simulink model "arduino_run"  (R2022a)
settings: Solver=FixedStepAuto  StartTime=0.0  StopTime=100  RelTol=1e-3  EnableMultiTasking=on
model workspace: external: MATLAB File D:\personal_projects\robot\biped-robot\robot_DataFile2.m (data not in the file)
libraries: arduinolib x48, simulink x12
settings Model: ExtModeTrigDuration=2  Creator=isamu  LastModifiedBy=isamu
settings OptimizationCC: EnhancedBackFolding=on  PassReuseOutputArgsAs=Individual arguments  ZeroExternalMemoryAtStartup=off  ZeroInternalMemoryAtStartup=off  MaxStackSize=64  OptimizeBlockOrder=speed  DifferentSizesBufferReuse=on  OptimizationCustomize=off  EfficientTunableParamExpr=on
settings DebuggingCC: ParameterTunabilityLossMsg=error
settings HardwareCC: ProdBitPerInt=16  ProdBitPerPointer=16  ProdBitPerSizeT=16  ProdBitPerPtrDiffT=16  ProdLargestAtomicFloat=None  ProdWordSize=8  ProdHWDeviceType=Atmel->AVR  UseEmbeddedCoderFeatures=off  UseSimulinkCoderFeatures=off
settings SFSimCC: MATLABDynamicMemAlloc=off
settings RTWCC: SystemTargetFile=ert.tlc  HardwareBoard=Arduino Mega 2560  TemplateMakefile=ert_default_tmf  Toolchain=Arduino AVR  BuildConfiguration=Faster Runs
settings CodeAppCC: ForceParamTrailComments=on  IgnoreCustomStorageClasses=off  OperatorAnnotations=on  SimulinkDataObjDesc=on  SFDataObjDesc=on  InsertBlockDesc=on
settings ERTTargetCC: SupportContinuousTime=on  SupportNonInlinedSFcns=on  SupportVariableSizeSignals=on  ExtModeTransport=3  ExtModeStaticAlloc=on  ExtModeStaticAllocSize=2048  ExtModeMexFile=ext_xcp  ExtModeIntrfLevel=Level2 - Open

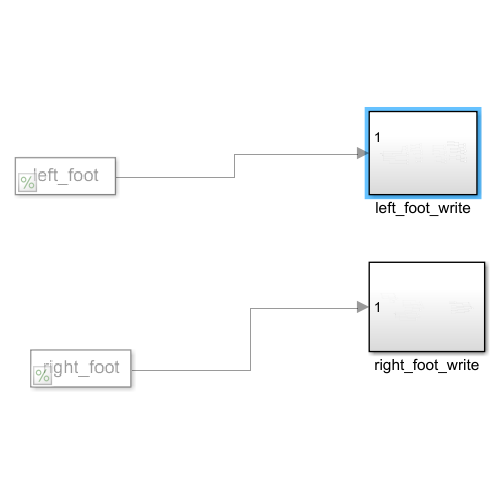
[thumbnail: Simulink's stored preview of the top-level diagram]
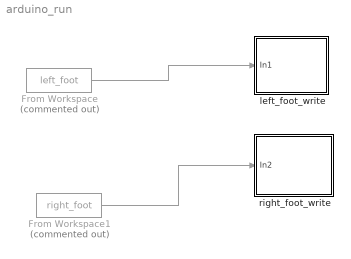
== system arduino_run ==
  From Workspace : FromWorkspace  Commented=on  VariableName=left_foot  OutDataTypeStr=Bus: left_foot_bus  SampleTime=0.045  OutputAfterFinalValue=Holding final value
  From Workspace1 : FromWorkspace  Commented=on  VariableName=right_foot  OutDataTypeStr=Bus: right_foot_bus  SampleTime=0.045  OutputAfterFinalValue=Holding final value
  left_foot_write : Subsystem
  right_foot_write : Subsystem
  wires:
  From Workspace/1 -> left_foot_write/1(In1)
  From Workspace1/1 -> right_foot_write/1(In2)

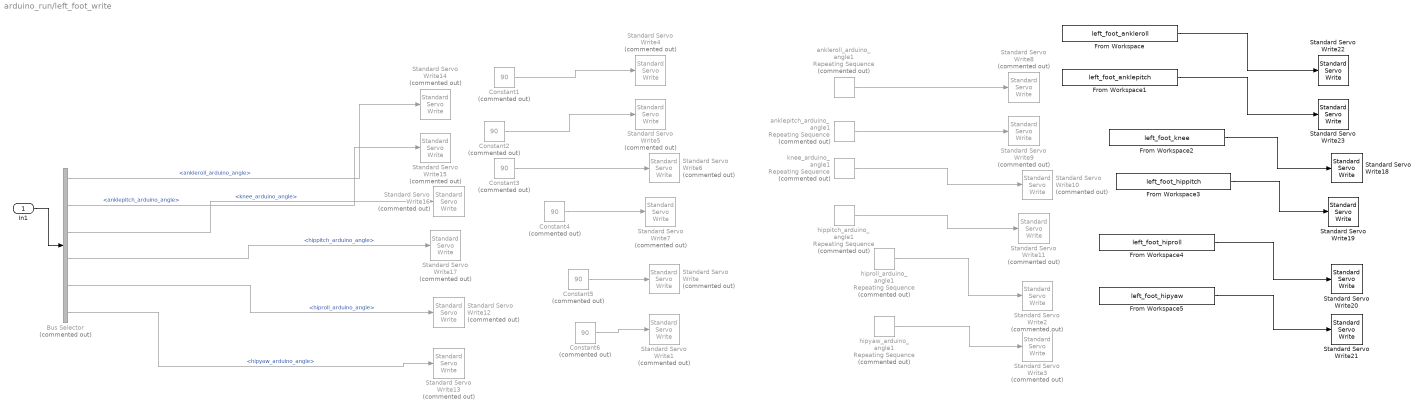
== system arduino_run/left_foot_write ==
  In1 : Inport
  Bus Selector : BusSelector  Commented=on  OutputSignals=ankleroll_arduino_angle,anklepitch_arduino_angle,knee_arduino_angle,hippitch_arduino_angle,hiproll_arduino_angle,hipyaw_arduino_angle
  Constant{1..6} (6 alike) : Constant  Commented=on  Value=90
  From Workspace : FromWorkspace  VariableName=left_foot_ankleroll  SampleTime=0.045  Interpolate=off  OutputAfterFinalValue=Cyclic repetition
  From Workspace1 : FromWorkspace  VariableName=left_foot_anklepitch  SampleTime=0.045  Interpolate=off  OutputAfterFinalValue=Cyclic repetition
  From Workspace2 : FromWorkspace  VariableName=left_foot_knee  SampleTime=0.045  Interpolate=off  OutputAfterFinalValue=Cyclic repetition
  From Workspace3 : FromWorkspace  VariableName=left_foot_hippitch  SampleTime=0.045  Interpolate=off  OutputAfterFinalValue=Cyclic repetition
  From Workspace4 : FromWorkspace  VariableName=left_foot_hiproll  SampleTime=0.045  Interpolate=off  OutputAfterFinalValue=Cyclic repetition
  From Workspace5 : FromWorkspace  VariableName=left_foot_hipyaw  SampleTime=0.045  Interpolate=off  OutputAfterFinalValue=Cyclic repetition
  Standard Servo Write : arduinolib/Standard Servo Write  Commented=on  pinNumber=12  ServoIndex=0  blockPlatform=ARDUINO
  Standard Servo Write1 : arduinolib/Standard Servo Write  Commented=on  pinNumber=13  ServoIndex=1  blockPlatform=ARDUINO
  Standard Servo Write10 : arduinolib/Standard Servo Write  Commented=on  pinNumber=10  ServoIndex=0  blockPlatform=ARDUINO
  Standard Servo Write11 : arduinolib/Standard Servo Write  Commented=on  pinNumber=11  ServoIndex=1  blockPlatform=ARDUINO
  Standard Servo Write12 : arduinolib/Standard Servo Write  Commented=on  pinNumber=12  ServoIndex=0  blockPlatform=ARDUINO
  Standard Servo Write13 : arduinolib/Standard Servo Write  Commented=on  pinNumber=13  ServoIndex=1  blockPlatform=ARDUINO
  Standard Servo Write14 : arduinolib/Standard Servo Write  Commented=on  pinNumber=8  ServoIndex=2  blockPlatform=ARDUINO
  Standard Servo Write15 : arduinolib/Standard Servo Write  Commented=on  pinNumber=9  ServoIndex=3  blockPlatform=ARDUINO
  Standard Servo Write16 : arduinolib/Standard Servo Write  Commented=on  pinNumber=10  ServoIndex=4  blockPlatform=ARDUINO
  Standard Servo Write17 : arduinolib/Standard Servo Write  Commented=on  pinNumber=11  ServoIndex=5  blockPlatform=ARDUINO
  Standard Servo Write18 : arduinolib/Standard Servo Write  pinNumber=10  ServoIndex=0  blockPlatform=ARDUINO
  Standard Servo Write19 : arduinolib/Standard Servo Write  pinNumber=11  ServoIndex=1  blockPlatform=ARDUINO
  Standard Servo Write2 : arduinolib/Standard Servo Write  Commented=on  pinNumber=12  ServoIndex=2  blockPlatform=ARDUINO
  Standard Servo Write20 : arduinolib/Standard Servo Write  pinNumber=12  ServoIndex=2  blockPlatform=ARDUINO
  Standard Servo Write21 : arduinolib/Standard Servo Write  pinNumber=13  ServoIndex=3  blockPlatform=ARDUINO
  Standard Servo Write22 : arduinolib/Standard Servo Write  pinNumber=8  ServoIndex=4  blockPlatform=ARDUINO
  Standard Servo Write23 : arduinolib/Standard Servo Write  pinNumber=9  ServoIndex=5  blockPlatform=ARDUINO
  Standard Servo Write3 : arduinolib/Standard Servo Write  Commented=on  pinNumber=13  ServoIndex=3  blockPlatform=ARDUINO
  Standard Servo Write4 : arduinolib/Standard Servo Write  Commented=on  pinNumber=8  ServoIndex=2  blockPlatform=ARDUINO
  Standard Servo Write5 : arduinolib/Standard Servo Write  Commented=on  pinNumber=9  ServoIndex=3  blockPlatform=ARDUINO
  Standard Servo Write6 : arduinolib/Standard Servo Write  Commented=on  pinNumber=10  ServoIndex=4  blockPlatform=ARDUINO
  Standard Servo Write7 : arduinolib/Standard Servo Write  Commented=on  pinNumber=11  ServoIndex=5  blockPlatform=ARDUINO
  Standard Servo Write8 : arduinolib/Standard Servo Write  Commented=on  pinNumber=8  ServoIndex=4  blockPlatform=ARDUINO
  Standard Servo Write9 : arduinolib/Standard Servo Write  Commented=on  pinNumber=9  ServoIndex=5  blockPlatform=ARDUINO
  anklepitch_arduino_angle1 : simulink/Sources/Repeating Sequence  Commented=on  rep_seq_t=robot_time  rep_seq_y=left_foot.anklepitch_arduino_angle.Data
  ankleroll_arduino_angle1 : simulink/Sources/Repeating Sequence  Commented=on  rep_seq_t=robot_time  rep_seq_y=left_foot.ankleroll_arduino_angle.Data
  hippitch_arduino_angle1 : simulink/Sources/Repeating Sequence  Commented=on  rep_seq_t=robot_time  rep_seq_y=left_foot.hippitch_arduino_angle.Data
  hiproll_arduino_angle1 : simulink/Sources/Repeating Sequence  Commented=on  rep_seq_t=robot_time  rep_seq_y=left_foot.hiproll_arduino_angle.Data
  hipyaw_arduino_angle1 : simulink/Sources/Repeating Sequence  Commented=on  rep_seq_t=robot_time  rep_seq_y=left_foot.hipyaw_arduino_angle.Data
  knee_arduino_angle1 : simulink/Sources/Repeating Sequence  Commented=on  rep_seq_t=robot_time  rep_seq_y=left_foot.knee_arduino_angle.Data
  wires:
  hippitch_arduino_angle1/1 -> Standard Servo Write11/1
  hipyaw_arduino_angle1/1 -> Standard Servo Write3/1
  hiproll_arduino_angle1/1 -> Standard Servo Write2/1
  anklepitch_arduino_angle1/1 -> Standard Servo Write9/1
  knee_arduino_angle1/1 -> Standard Servo Write10/1
  ankleroll_arduino_angle1/1 -> Standard Servo Write8/1
  Constant1/1 -> Standard Servo Write4/1
  Constant2/1 -> Standard Servo Write5/1
  Constant3/1 -> Standard Servo Write6/1
  Constant4/1 -> Standard Servo Write7/1
  Constant5/1 -> Standard Servo Write/1
  Constant6/1 -> Standard Servo Write1/1
  In1/1 -> Bus Selector/1
  Bus Selector/1 -> Standard Servo Write14/1  "<ankleroll_arduino_angle>"
  Bus Selector/2 -> Standard Servo Write15/1  "<anklepitch_arduino_angle>"
  Bus Selector/3 -> Standard Servo Write16/1  "<knee_arduino_angle>"
  Bus Selector/4 -> Standard Servo Write17/1  "<hippitch_arduino_angle>"
  Bus Selector/5 -> Standard Servo Write12/1  "<hiproll_arduino_angle>"
  Bus Selector/6 -> Standard Servo Write13/1  "<hipyaw_arduino_angle>"
  From Workspace/1 -> Standard Servo Write22/1
  From Workspace1/1 -> Standard Servo Write23/1
  From Workspace2/1 -> Standard Servo Write18/1
  From Workspace3/1 -> Standard Servo Write19/1
  From Workspace4/1 -> Standard Servo Write20/1
  From Workspace5/1 -> Standard Servo Write21/1

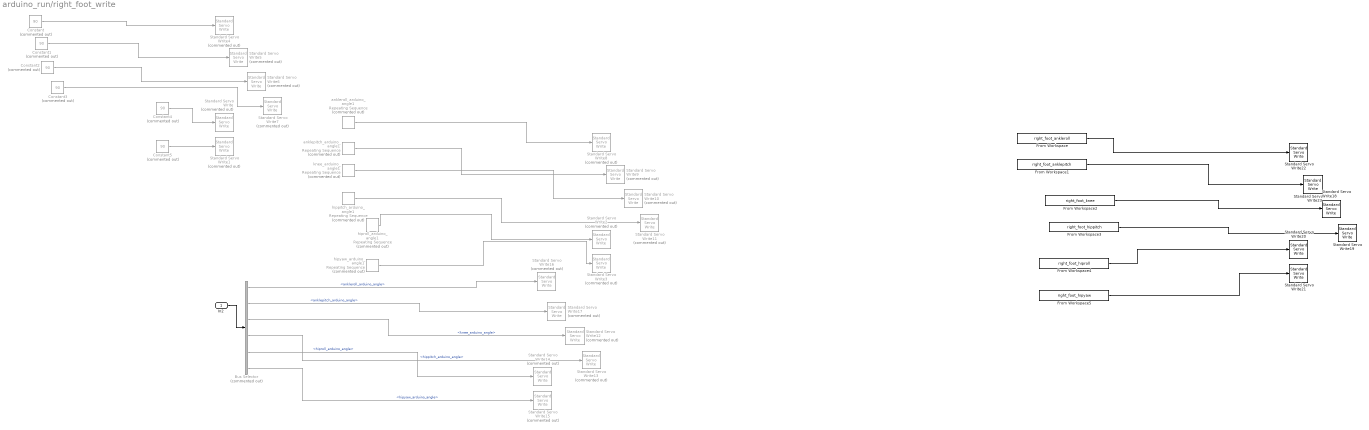
== system arduino_run/right_foot_write ==
  In2 : Inport
  Bus Selector : BusSelector  Commented=on  OutputSignals=ankleroll_arduino_angle,anklepitch_arduino_angle,knee_arduino_angle,hippitch_arduino_angle,hiproll_arduino_angle,hipyaw_arduino_angle
  Constant{,1..5} (6 alike) : Constant  Commented=on  Value=90
  From Workspace : FromWorkspace  VariableName=right_foot_ankleroll  SampleTime=0.045  Interpolate=off  OutputAfterFinalValue=Cyclic repetition
  From Workspace1 : FromWorkspace  VariableName=right_foot_anklepitch  SampleTime=0.045  Interpolate=off  OutputAfterFinalValue=Cyclic repetition
  From Workspace2 : FromWorkspace  VariableName=right_foot_knee  SampleTime=0.045  Interpolate=off  OutputAfterFinalValue=Cyclic repetition
  From Workspace3 : FromWorkspace  VariableName=right_foot_hippitch  SampleTime=0.045  Interpolate=off  OutputAfterFinalValue=Cyclic repetition
  From Workspace4 : FromWorkspace  VariableName=right_foot_hiproll  SampleTime=0.045  Interpolate=off  OutputAfterFinalValue=Cyclic repetition
  From Workspace5 : FromWorkspace  VariableName=right_foot_hipyaw  SampleTime=0.045  Interpolate=off  OutputAfterFinalValue=Cyclic repetition
  Standard Servo Write : arduinolib/Standard Servo Write  Commented=on  pinNumber=6  ServoIndex=6  blockPlatform=ARDUINO
  Standard Servo Write1 : arduinolib/Standard Servo Write  Commented=on  pinNumber=7  ServoIndex=7  blockPlatform=ARDUINO
  Standard Servo Write10 : arduinolib/Standard Servo Write  Commented=on  pinNumber=4  ServoIndex=6  blockPlatform=ARDUINO
  Standard Servo Write11 : arduinolib/Standard Servo Write  Commented=on  pinNumber=5  ServoIndex=7  blockPlatform=ARDUINO
  Standard Servo Write12 : arduinolib/Standard Servo Write  Commented=on  pinNumber=4  ServoIndex=6  blockPlatform=ARDUINO
  Standard Servo Write13 : arduinolib/Standard Servo Write  Commented=on  pinNumber=5  ServoIndex=7  blockPlatform=ARDUINO
  Standard Servo Write14 : arduinolib/Standard Servo Write  Commented=on  pinNumber=6  ServoIndex=8  blockPlatform=ARDUINO
  Standard Servo Write15 : arduinolib/Standard Servo Write  Commented=on  pinNumber=7  ServoIndex=9  blockPlatform=ARDUINO
  Standard Servo Write16 : arduinolib/Standard Servo Write  Commented=on  pinNumber=2  ServoIndex=10  blockPlatform=ARDUINO
  Standard Servo Write17 : arduinolib/Standard Servo Write  Commented=on  pinNumber=3  ServoIndex=11  blockPlatform=ARDUINO
  Standard Servo Write18 : arduinolib/Standard Servo Write  pinNumber=4  ServoIndex=6  blockPlatform=ARDUINO
  Standard Servo Write19 : arduinolib/Standard Servo Write  pinNumber=5  ServoIndex=7  blockPlatform=ARDUINO
  Standard Servo Write2 : arduinolib/Standard Servo Write  Commented=on  pinNumber=6  ServoIndex=8  blockPlatform=ARDUINO
  Standard Servo Write20 : arduinolib/Standard Servo Write  pinNumber=6  ServoIndex=8  blockPlatform=ARDUINO
  Standard Servo Write21 : arduinolib/Standard Servo Write  pinNumber=7  ServoIndex=9  blockPlatform=ARDUINO
  Standard Servo Write22 : arduinolib/Standard Servo Write  pinNumber=2  ServoIndex=10  blockPlatform=ARDUINO
  Standard Servo Write23 : arduinolib/Standard Servo Write  pinNumber=3  ServoIndex=11  blockPlatform=ARDUINO
  Standard Servo Write3 : arduinolib/Standard Servo Write  Commented=on  pinNumber=7  ServoIndex=9  blockPlatform=ARDUINO
  Standard Servo Write4 : arduinolib/Standard Servo Write  Commented=on  pinNumber=2  ServoIndex=8  blockPlatform=ARDUINO
  Standard Servo Write5 : arduinolib/Standard Servo Write  Commented=on  pinNumber=3  ServoIndex=9  blockPlatform=ARDUINO
  Standard Servo Write6 : arduinolib/Standard Servo Write  Commented=on  pinNumber=4  ServoIndex=10  blockPlatform=ARDUINO
  Standard Servo Write7 : arduinolib/Standard Servo Write  Commented=on  pinNumber=5  ServoIndex=11  blockPlatform=ARDUINO
  Standard Servo Write8 : arduinolib/Standard Servo Write  Commented=on  pinNumber=2  ServoIndex=10  blockPlatform=ARDUINO
  Standard Servo Write9 : arduinolib/Standard Servo Write  Commented=on  pinNumber=3  ServoIndex=11  blockPlatform=ARDUINO
  anklepitch_arduino_angle1 : simulink/Sources/Repeating Sequence  Commented=on  rep_seq_t=robot_time  rep_seq_y=right_foot.anklepitch_arduino_angle.Data
  ankleroll_arduino_angle1 : simulink/Sources/Repeating Sequence  Commented=on  rep_seq_t=robot_time  rep_seq_y=right_foot.ankleroll_arduino_angle.Data
  hippitch_arduino_angle1 : simulink/Sources/Repeating Sequence  Commented=on  rep_seq_t=robot_time  rep_seq_y=right_foot.hippitch_arduino_angle.Data
  hiproll_arduino_angle1 : simulink/Sources/Repeating Sequence  Commented=on  rep_seq_t=robot_time  rep_seq_y=right_foot.hiproll_arduino_angle.Data
  hipyaw_arduino_angle1 : simulink/Sources/Repeating Sequence  Commented=on  rep_seq_t=robot_time  rep_seq_y=right_foot.hipyaw_arduino_angle.Data
  knee_arduino_angle1 : simulink/Sources/Repeating Sequence  Commented=on  rep_seq_t=robot_time  rep_seq_y=right_foot.knee_arduino_angle.Data
  wires:
  knee_arduino_angle1/1 -> Standard Servo Write10/1
  hiproll_arduino_angle1/1 -> Standard Servo Write2/1
  hippitch_arduino_angle1/1 -> Standard Servo Write11/1
  anklepitch_arduino_angle1/1 -> Standard Servo Write9/1
  ankleroll_arduino_angle1/1 -> Standard Servo Write8/1
  hipyaw_arduino_angle1/1 -> Standard Servo Write3/1
  Constant/1 -> Standard Servo Write4/1
  Constant1/1 -> Standard Servo Write5/1
  Constant2/1 -> Standard Servo Write6/1
  Constant3/1 -> Standard Servo Write7/1
  Constant4/1 -> Standard Servo Write/1
  Constant5/1 -> Standard Servo Write1/1
  Bus Selector/6 -> Standard Servo Write15/1  "<hipyaw_arduino_angle>"
  Bus Selector/2 -> Standard Servo Write17/1  "<anklepitch_arduino_angle>"
  Bus Selector/1 -> Standard Servo Write16/1  "<ankleroll_arduino_angle>"
  Bus Selector/4 -> Standard Servo Write13/1  "<hippitch_arduino_angle>"
  Bus Selector/3 -> Standard Servo Write12/1  "<knee_arduino_angle>"
  Bus Selector/5 -> Standard Servo Write14/1  "<hiproll_arduino_angle>"
  In2/1 -> Bus Selector/1
  From Workspace1/1 -> Standard Servo Write23/1
  From Workspace5/1 -> Standard Servo Write21/1
  From Workspace/1 -> Standard Servo Write22/1
  From Workspace4/1 -> Standard Servo Write20/1
  From Workspace2/1 -> Standard Servo Write18/1
  From Workspace3/1 -> Standard Servo Write19/1
